simulink model "SEMINAR_DFIG_RSC_Controller"  (R2014a)
settings: Solver=ode45  StartTime=0.0  StopTime=10.0  RelTol=1e-3
libraries: powerlib_meascontrol x7, simulink x3, powerlib x1
settings Model: Creator=ninad gaikawad  LastModifiedBy=ninad gaikawad

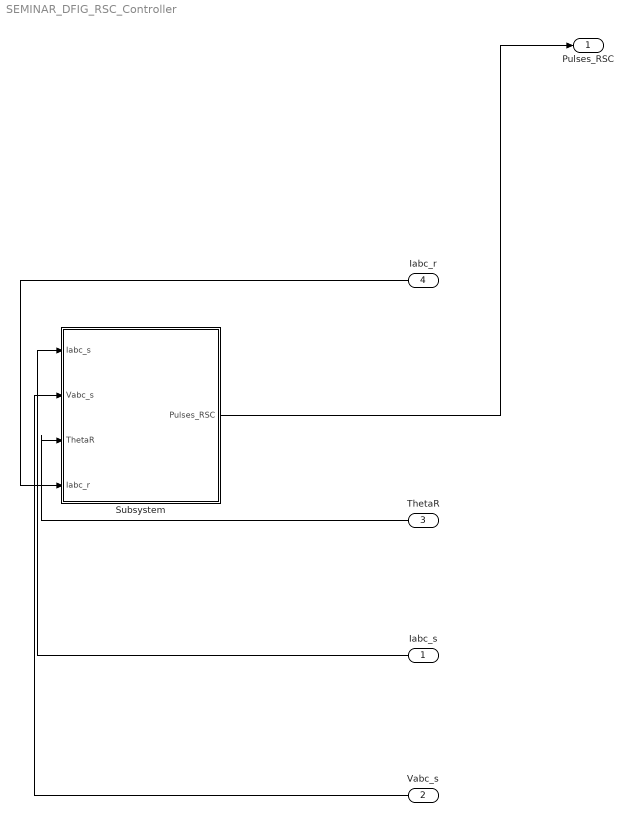
== system SEMINAR_DFIG_RSC_Controller ==
  Iabc_s : Inport
  Vabc_s : Inport  Port=2
  ThetaR : Inport  Port=3
  Iabc_r : Inport  Port=4
  Subsystem : Subsystem
  Pulses_RSC : Outport
  wires:
  Iabc_s/1 -> Subsystem/1(Iabc_s)
  Vabc_s/1 -> Subsystem/2(Vabc_s)
  ThetaR/1 -> Subsystem/3(ThetaR)
  Iabc_r/1 -> Subsystem/4(Iabc_r)
  Subsystem/1(Pulses_RSC) -> Pulses_RSC/1

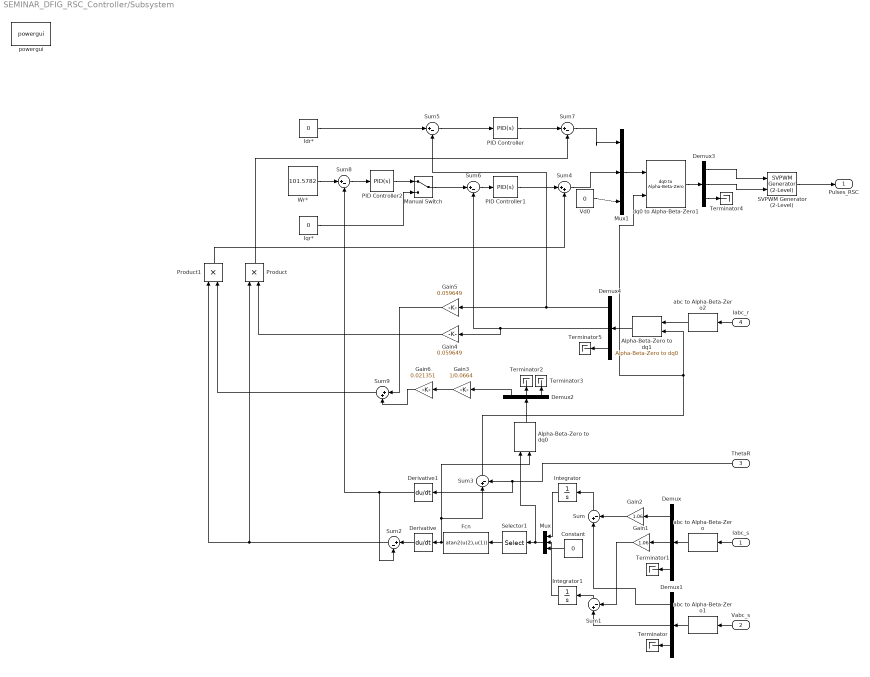
== system SEMINAR_DFIG_RSC_Controller/Subsystem ==
  Iabc_s : Inport
  Vabc_s : Inport  Port=2
  ThetaR : Inport  Port=3
  Iabc_r : Inport  Port=4
  Alpha-Beta-Zero to dq0 : powerlib_meascontrol/Transformations/Alpha-Beta-Zero to dq0  Alignment=90 degrees behind phase A axis
  Alpha-Beta-Zero to dq1 : powerlib_meascontrol/Transformations/Alpha-Beta-Zero to dq0  Alignment=90 degrees behind phase A axis
  Constant : Constant  Value=0
  Demux{,1..4} (5 alike) : Demux  Outputs=3
  Derivative : Derivative
  Derivative1 : Derivative
  Fcn : Fcn  Expr=atan2(u(2),u(1))
  Gain1 : Gain  Gain=1.06
  Gain2 : Gain  Gain=1.06
  Gain3 : Gain  Gain=1/0.0664
  Gain4 : Gain  Gain=0.059649
  Gain5 : Gain  Gain=0.059649
  Gain6 : Gain  Gain=0.021351
  Idr* : Constant  Value=0
  Integrator : Integrator
  Integrator1 : Integrator
  Iqr* : Constant  Value=0
  Manual Switch : ManualSwitch
  Mux : Mux  Inputs=3
  Mux1 : Mux  Inputs=3
  PID Controller : simulink/Continuous/PID Controller  Controller=PID  TimeDomain=Continuous-time  SampleTime=1  IntegratorMethod=Forward Euler  FilterMethod=Forward Euler  Form=Parallel  P=1  I=1  D=0  N=100  InitialConditionSource=internal  InitialConditionForIntegrator=0  InitialConditionForFilter=0  ExternalReset=none  LimitOutput=off  UpperSaturationLimit=inf  LowerSaturationLimit=-inf  LinearizeAsGain=on  AntiWindupMode=none  Kb=1  TrackingMode=off  Kt=1  PParamMin=[]  PParamMax=[]  IParamMin=[]  IParamMax=[]  DParamMin=[]  DParamMax=[]  NParamMin=[]  NParamMax=[]  KbParamMin=[]  KbParamMax=[]  KtParamMin=[]  KtParamMax=[]  POutMin=[]  POutMax=[]  IOutMin=[]  IOutMax=[]  DOutMin=[]  DOutMax=[]  NOutMin=[]  NOutMax=[]  KbOutMin=[]  KbOutMax=[]  KtOutMin=[]  KtOutMax=[]  IntegratorOutMin=[]  IntegratorOutMax=[]  FilterOutMin=[]  FilterOutMax=[]  SumOutMin=[]  SumOutMax=[]  SumI1OutMin=[]  SumI1OutMax=[]  SumI2OutMin=[]  SumI2OutMax=[]  SumI3OutMin=[]  SumI3OutMax=[]  SumDOutMin=[]  SumDOutMax=[]  SaturationOutMin=[]  SaturationOutMax=[]  IntegratorContinuousStateAttributes=''  IntegratorStateMustResolveToSignalObject=off  IntegratorRTWStateStorageClass=Auto  FilterContinuousStateAttributes=''  FilterStateMustResolveToSignalObject=off  FilterRTWStateStorageClass=Auto
  PID Controller1 : simulink/Continuous/PID Controller  Controller=PID  TimeDomain=Continuous-time  SampleTime=1  IntegratorMethod=Forward Euler  FilterMethod=Forward Euler  Form=Parallel  P=1  I=1  D=0  N=100  InitialConditionSource=internal  InitialConditionForIntegrator=0  InitialConditionForFilter=0  ExternalReset=none  LimitOutput=off  UpperSaturationLimit=inf  LowerSaturationLimit=-inf  LinearizeAsGain=on  AntiWindupMode=none  Kb=1  TrackingMode=off  Kt=1  PParamMin=[]  PParamMax=[]  IParamMin=[]  IParamMax=[]  DParamMin=[]  DParamMax=[]  NParamMin=[]  NParamMax=[]  KbParamMin=[]  KbParamMax=[]  KtParamMin=[]  KtParamMax=[]  POutMin=[]  POutMax=[]  IOutMin=[]  IOutMax=[]  DOutMin=[]  DOutMax=[]  NOutMin=[]  NOutMax=[]  KbOutMin=[]  KbOutMax=[]  KtOutMin=[]  KtOutMax=[]  IntegratorOutMin=[]  IntegratorOutMax=[]  FilterOutMin=[]  FilterOutMax=[]  SumOutMin=[]  SumOutMax=[]  SumI1OutMin=[]  SumI1OutMax=[]  SumI2OutMin=[]  SumI2OutMax=[]  SumI3OutMin=[]  SumI3OutMax=[]  SumDOutMin=[]  SumDOutMax=[]  SaturationOutMin=[]  SaturationOutMax=[]  IntegratorContinuousStateAttributes=''  IntegratorStateMustResolveToSignalObject=off  IntegratorRTWStateStorageClass=Auto  FilterContinuousStateAttributes=''  FilterStateMustResolveToSignalObject=off  FilterRTWStateStorageClass=Auto
  PID Controller2 : simulink/Continuous/PID Controller  Controller=PID  TimeDomain=Continuous-time  SampleTime=1  IntegratorMethod=Forward Euler  FilterMethod=Forward Euler  Form=Parallel  P=1  I=1  D=0  N=100  InitialConditionSource=internal  InitialConditionForIntegrator=0  InitialConditionForFilter=0  ExternalReset=none  LimitOutput=off  UpperSaturationLimit=inf  LowerSaturationLimit=-inf  LinearizeAsGain=on  AntiWindupMode=none  Kb=1  TrackingMode=off  Kt=1  PParamMin=[]  PParamMax=[]  IParamMin=[]  IParamMax=[]  DParamMin=[]  DParamMax=[]  NParamMin=[]  NParamMax=[]  KbParamMin=[]  KbParamMax=[]  KtParamMin=[]  KtParamMax=[]  POutMin=[]  POutMax=[]  IOutMin=[]  IOutMax=[]  DOutMin=[]  DOutMax=[]  NOutMin=[]  NOutMax=[]  KbOutMin=[]  KbOutMax=[]  KtOutMin=[]  KtOutMax=[]  IntegratorOutMin=[]  IntegratorOutMax=[]  FilterOutMin=[]  FilterOutMax=[]  SumOutMin=[]  SumOutMax=[]  SumI1OutMin=[]  SumI1OutMax=[]  SumI2OutMin=[]  SumI2OutMax=[]  SumI3OutMin=[]  SumI3OutMax=[]  SumDOutMin=[]  SumDOutMax=[]  SaturationOutMin=[]  SaturationOutMax=[]  IntegratorContinuousStateAttributes=''  IntegratorStateMustResolveToSignalObject=off  IntegratorRTWStateStorageClass=Auto  FilterContinuousStateAttributes=''  FilterStateMustResolveToSignalObject=off  FilterRTWStateStorageClass=Auto
  Product : Product
  Product1 : Product
  SVPWM Generator (2-Level) : powerlib_meascontrol/Pulse & Signal Generators/SVPWM Generator (2-Level)  InputType=alpha-beta components  SwitchingPattern=Pattern #1  Fc=27*50  ParUref=[0.8 -30 50]  Ts=0
  Selector1 : Selector  InputPortWidth=3  Indices=[1 2]
  Sum{,1..3,5..8} (8 alike) : Sum  Inputs=|+-
  Sum4 : Sum  Inputs=|++
  Sum9 : Sum  Inputs=|++
  Terminator{,1..5} (6 alike) : Terminator
  Vd0 : Constant  Value=0
  Wr* : Constant  Value=101.5782
  abc to Alpha-Beta-Zero : powerlib_meascontrol/Transformations/abc to Alpha-Beta-Zero
  abc to Alpha-Beta-Zero1 : powerlib_meascontrol/Transformations/abc to Alpha-Beta-Zero
  abc to Alpha-Beta-Zero2 : powerlib_meascontrol/Transformations/abc to Alpha-Beta-Zero
  dq0 to Alpha-Beta-Zero1 : powerlib_meascontrol/Transformations/dq0 to Alpha-Beta-Zero  Alignment=90 degrees behind phase A axis
  powergui : powerlib/powergui  Priority=1  SimulationMode=Continuous  SolverType=Tustin  SampleTime=50e-6  frequency=60  SPID=off  DisableSnubberDevices=off  DisableRonSwitches=off  DisableVfSwitches=off  SwTol=0  Interpol=off  DisplayEquations=off  Ts=0  methode=off  frequencyindice=60  Pbase=100e6  ErrMax=1e-4  Iterations=50  UnitsV=kV  UnitsW=MW  FunctionMessages=off  echomessages=off  HookPort=off  EnableUseOfTLC=off  x0status=blocks  RestoreLinks=warning  ResistiveCurrentMeasurement=off  Frange=[0:2:500]  Ylog=off  Xlog=on  ShowGrid=off  save=off  variable=ZData  structure=0  ZoomFFT=off  StartTime=0.0  cycles=1  DisplayStyle=1  fundamental=60  FreqAxis=off  MaxFrequency=1000  frequencyindicesteady=1  RmsSteady=1  display=off
  Pulses_RSC : Outport
  wires:
  Gain2/1 -> Sum/2
  Sum/1 -> Integrator/1
  Demux/2 -> Gain1/1
  Demux1/2 -> Sum1/1
  Demux/1 -> Gain2/1
  Demux1/1 -> Sum/1
  SVPWM Generator (2-Level)/1 -> Pulses_RSC/1
  dq0 to Alpha-Beta-Zero1/1 -> Demux3/1
  Demux3/1 -> SVPWM Generator (2-Level)/1
  Demux3/3 -> Terminator4/1
  Demux3/2 -> SVPWM Generator (2-Level)/2
  Vabc_s/1 -> abc to Alpha-Beta-Zero1/1
  Iabc_s/1 -> abc to Alpha-Beta-Zero/1
  Integrator1/1 -> Mux/2
  Constant/1 -> Mux/3
  Selector1/1 -> Fcn/1
  Sum1/1 -> Integrator1/1
  ThetaR/1 -> Derivative1/1, Sum3/2
  Gain4/1 -> Product/2
  Mux/1 -> Alpha-Beta-Zero to dq0/1, Selector1/1
  Gain1/1 -> Sum1/2
  Integrator/1 -> Mux/1
  Fcn/1 -> Sum3/1, Alpha-Beta-Zero to dq0/2, Derivative/1
  Derivative/1 -> Sum2/1
  Sum2/1 -> Product1/1, Product/1
  Demux4/1 -> Sum5/2, Gain5/1
  Demux4/2 -> Gain4/1, Sum6/2
  Demux4/3 -> Terminator5/1
  Sum8/1 -> PID Controller2/1
  Derivative1/1 -> Sum8/2, Sum2/2
  Wr*/1 -> Sum8/1
  Gain3/1 -> Gain6/1
  Alpha-Beta-Zero to dq1/1 -> Demux4/1
  Alpha-Beta-Zero to dq0/1 -> Demux2/1
  Sum3/1 -> dq0 to Alpha-Beta-Zero1/2, Alpha-Beta-Zero to dq1/2
  Product1/1 -> Sum4/2
  abc to Alpha-Beta-Zero2/1 -> Alpha-Beta-Zero to dq1/1
  Mux1/1 -> dq0 to Alpha-Beta-Zero1/1
  Sum7/1 -> Mux1/1
  Vd0/1 -> Mux1/3
  Demux2/3 -> Terminator3/1
  PID Controller1/1 -> Sum4/1
  Demux2/2 -> Terminator2/1
  Demux2/1 -> Gain3/1
  Iabc_r/1 -> abc to Alpha-Beta-Zero2/1
  Product/1 -> Sum7/2
  Sum4/1 -> Mux1/2
  Idr*/1 -> Sum5/1
  Sum5/1 -> PID Controller/1
  Sum9/1 -> Product1/2
  Iqr*/1 -> Manual Switch/2
  Gain6/1 -> Sum9/2
  Manual Switch/1 -> Sum6/1
  PID Controller/1 -> Sum7/1
  Gain5/1 -> Sum9/1
  abc to Alpha-Beta-Zero1/1 -> Demux1/1
  abc to Alpha-Beta-Zero/1 -> Demux/1
  Sum6/1 -> PID Controller1/1
  PID Controller2/1 -> Manual Switch/1
  Demux/3 -> Terminator1/1
  Demux1/3 -> Terminator/1
